simulink model "LinearRegressorIP"  (R2022b)
settings: Solver=VariableStepAuto  StartTime=0.0  StopTime=StopTime  RelTol=1e-3
values from neighbouring files (symbols this model uses):
  ADC_SampleTime = 1/ADC_Freq    (= 1e-06)    [LR_Init.m]
  Harmonics_Power = 1/2    (= 0.5)    [LR_Init.m]
  Noise_SampleTime = ADC_SampleTime    (= 1e-06)    [LR_Init.m]
  Noise_Source = 4    [LR_Init.m]
  Signal_Amp = 35    [LR_Init.m]
  Signal_Freq = 333    [LR_Init.m]
  Signal_Phase = pi/2    (= 1.57079632679)    [LR_Init.m]
  Spike_Level_min = 10    [LR_Init.m]
libraries: simulink x2
settings Model: Creator=Admin  LastModifiedBy=Admin

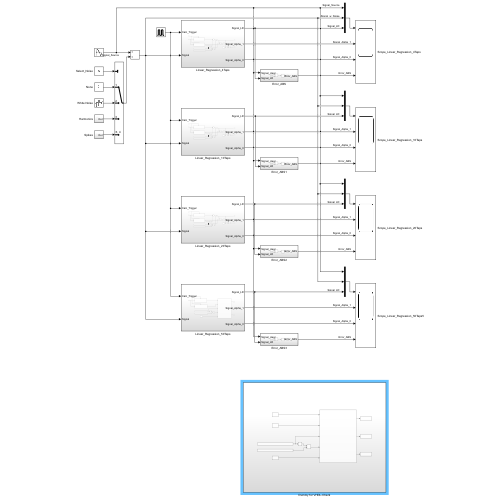
[thumbnail: Simulink's stored preview of the top-level diagram]
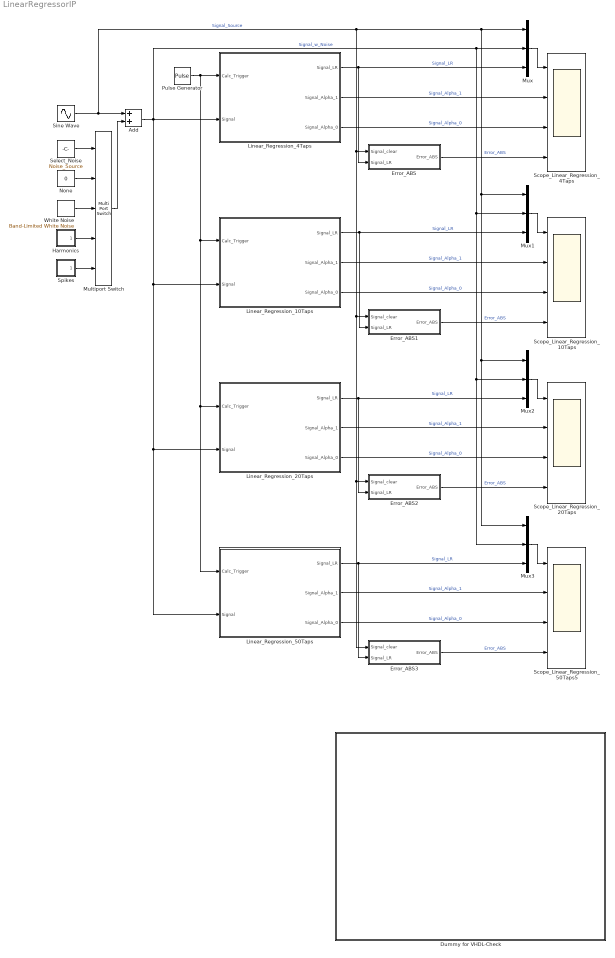
== system LinearRegressorIP ==
  Add : Sum
  Dummy for VHDL-Check : Subsystem
  Error_ABS : Subsystem
  Error_ABS1 : Subsystem
  Error_ABS2 : Subsystem
  Error_ABS3 : Subsystem
  Harmonics : Subsystem
  Linear_Regression_10Taps : Subsystem
  Linear_Regression_20Taps : Subsystem
  Linear_Regression_4Taps : Subsystem
  Linear_Regression_50Taps : Subsystem
  Multiport Switch : MultiPortSwitch  Inputs=4  SaturateOnIntegerOverflow=off  InputSameDT=off
  Mux{,1..3} (4 alike) : Mux  Inputs=3
  None : Constant  Value=0
  Pulse Generator : DiscretePulseGenerator  PulseType=Time based  Period=ADC_SampleTime  PulseWidth=50
  Scope_Linear_Regression_10Taps : Scope  NumInputPorts=4
  Scope_Linear_Regression_20Taps : Scope  NumInputPorts=4
  Scope_Linear_Regression_4Taps : Scope  NumInputPorts=4
  Scope_Linear_Regression_50Taps5 : Scope  NumInputPorts=4
  Select_Noise : Constant  Value=Noise_Source
  Sine Wave : Sin  Amplitude=Signal_Amp  Frequency=Signal_Freq*2*pi  Phase=Signal_Phase  SampleTime=0
  Spikes : Subsystem
  White Noise : simulink/Sources/Band-Limited White Noise  Cov=Noise_Power  Ts=Noise_SampleTime  seed=Noise_Seed
  wires:
  Pulse Generator/1 -> Linear_Regression_4Taps/1(Calc_Trigger), Linear_Regression_20Taps/1(Calc_Trigger), Linear_Regression_50Taps/1(Calc_Trigger), Linear_Regression_10Taps/1(Calc_Trigger)
  Sine Wave/1 -> Mux/1, Mux2/1, Mux3/1, Mux1/1, Error_ABS1/1(Signal_clear), Error_ABS3/1(Signal_clear), Error_ABS2/1(Signal_clear), Error_ABS/1(Signal_clear), Add/1  "Signal_Source"
  Multiport Switch/1 -> Add/2
  Add/1 -> Linear_Regression_4Taps/2(Signal), Linear_Regression_50Taps/2(Signal), Linear_Regression_20Taps/2(Signal), Linear_Regression_10Taps/2(Signal), Mux3/2, Mux2/2, Mux1/2, Mux/2  "Signal_w_Noise"
  Linear_Regression_4Taps/1(Signal_LR) -> Error_ABS/2(Signal_LR), Mux/3  "Signal_LR"
  Mux/1 -> Scope_Linear_Regression_4Taps/1
  Linear_Regression_4Taps/2(Signal_Alpha_1) -> Scope_Linear_Regression_4Taps/2  "Signal_Alpha_1"
  Linear_Regression_4Taps/3(Signal_Alpha_0) -> Scope_Linear_Regression_4Taps/3  "Signal_Alpha_0"
  Linear_Regression_10Taps/3(Signal_Alpha_0) -> Scope_Linear_Regression_10Taps/3  "Signal_Alpha_0"
  Linear_Regression_10Taps/2(Signal_Alpha_1) -> Scope_Linear_Regression_10Taps/2  "Signal_Alpha_1"
  Mux1/1 -> Scope_Linear_Regression_10Taps/1
  Linear_Regression_10Taps/1(Signal_LR) -> Error_ABS1/2(Signal_LR), Mux1/3  "Signal_LR"
  Mux2/1 -> Scope_Linear_Regression_20Taps/1
  Linear_Regression_20Taps/3(Signal_Alpha_0) -> Scope_Linear_Regression_20Taps/3  "Signal_Alpha_0"
  Linear_Regression_20Taps/2(Signal_Alpha_1) -> Scope_Linear_Regression_20Taps/2  "Signal_Alpha_1"
  Linear_Regression_20Taps/1(Signal_LR) -> Error_ABS2/2(Signal_LR), Mux2/3  "Signal_LR"
  Linear_Regression_50Taps/2(Signal_Alpha_1) -> Scope_Linear_Regression_50Taps5/2  "Signal_Alpha_1"
  Linear_Regression_50Taps/1(Signal_LR) -> Error_ABS3/2(Signal_LR), Mux3/3  "Signal_LR"
  Mux3/1 -> Scope_Linear_Regression_50Taps5/1
  Linear_Regression_50Taps/3(Signal_Alpha_0) -> Scope_Linear_Regression_50Taps5/3  "Signal_Alpha_0"
  Error_ABS/1(Error_ABS) -> Scope_Linear_Regression_4Taps/4  "Error_ABS"
  Error_ABS1/1(Error_ABS) -> Scope_Linear_Regression_10Taps/4  "Error_ABS"
  Error_ABS2/1(Error_ABS) -> Scope_Linear_Regression_20Taps/4  "Error_ABS"
  Error_ABS3/1(Error_ABS) -> Scope_Linear_Regression_50Taps5/4  "Error_ABS"
  Select_Noise/1 -> Multiport Switch/1
  None/1 -> Multiport Switch/2
  White Noise/1 -> Multiport Switch/3
  Harmonics/1(Out) -> Multiport Switch/4
  Spikes/1(Out) -> Multiport Switch/5

== system LinearRegressorIP/Dummy for VHDL-Check ==
  Constant : Constant  Value=50
  Constant3 : Constant  Value=25.5
  Constant4 : Constant  Value=858.5
  Constant5 : Constant
  LR_Calcer : Subsystem
  Pulse Generator : DiscretePulseGenerator  PulseType=Time based  Period=ADC_SampleTime  PulseWidth=50
  Running_mean_Window_50_Signal : Subsystem
  Running_mean_Window_50_SignalTimesSample : Subsystem
  Scope : Scope
  Scope1 : Scope
  Scope2 : Scope  NumInputPorts=3
  Square : Math  Operator=square
  Subtract1 : Sum  Inputs=-+
  wires:
  Subtract1/1 -> LR_Calcer/4(FaktorCalcAlpha1)
  Constant/1 -> LR_Calcer/5(Tabs)
  Constant4/1 -> Subtract1/2
  Constant3/1 -> Square/1, LR_Calcer/3(samples_mean)
  Square/1 -> Subtract1/1
  LR_Calcer/3(Signal_LR) -> Scope2/3  "Signal_LR"
  Running_mean_Window_50_SignalTimesSample/1(Signal_Output_Mean) -> LR_Calcer/1(RMW_SignalTimesSample), Scope/1
  Running_mean_Window_50_Signal/1(Signal_Output_Mean) -> LR_Calcer/2(RMW_Signal), Scope1/1
  Pulse Generator/1 -> Running_mean_Window_50_Signal/Trigger, Running_mean_Window_50_SignalTimesSample/Trigger
  Constant5/1 -> Running_mean_Window_50_SignalTimesSample/1(Signal_Input), Running_mean_Window_50_Signal/1(Signal_Input)
  LR_Calcer/1(Alpha_1) -> Scope2/1  "Alpha_1"
  LR_Calcer/2(Alpha_0) -> Scope2/2  "Alpha_0"

== system LinearRegressorIP/Error_ABS ==
  Signal_clear : Inport
  Signal_LR : Inport  Port=2
  Abs : Abs  SaturateOnIntegerOverflow=off
  Subtract : Sum  Inputs=+-
  Error_ABS : Outport
  wires:
  Abs/1 -> Error_ABS/1
  Subtract/1 -> Abs/1
  Signal_clear/1 -> Subtract/1
  Signal_LR/1 -> Subtract/2

== system LinearRegressorIP/Error_ABS1 ==
  Signal_clear : Inport
  Signal_LR : Inport  Port=2
  Abs : Abs  SaturateOnIntegerOverflow=off
  Subtract : Sum  Inputs=+-
  Error_ABS : Outport
  wires:
  Signal_LR/1 -> Subtract/2
  Signal_clear/1 -> Subtract/1
  Subtract/1 -> Abs/1
  Abs/1 -> Error_ABS/1

== system LinearRegressorIP/Error_ABS2 ==
  Signal_clear : Inport
  Signal_LR : Inport  Port=2
  Abs : Abs  SaturateOnIntegerOverflow=off
  Subtract : Sum  Inputs=+-
  Error_ABS : Outport
  wires:
  Abs/1 -> Error_ABS/1
  Subtract/1 -> Abs/1
  Signal_clear/1 -> Subtract/1
  Signal_LR/1 -> Subtract/2

== system LinearRegressorIP/Error_ABS3 ==
  Signal_clear : Inport
  Signal_LR : Inport  Port=2
  Abs : Abs  SaturateOnIntegerOverflow=off
  Subtract : Sum  Inputs=+-
  Error_ABS : Outport
  wires:
  Signal_LR/1 -> Subtract/2
  Signal_clear/1 -> Subtract/1
  Subtract/1 -> Abs/1
  Abs/1 -> Error_ABS/1

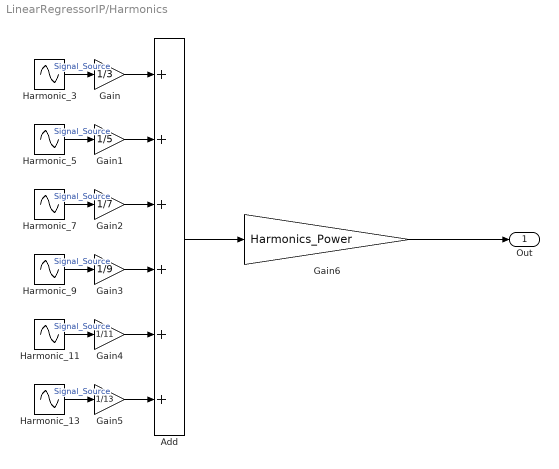
== system LinearRegressorIP/Harmonics ==
  Add : Sum  Inputs=++++++
  Gain : Gain  Gain=1/3
  Gain1 : Gain  Gain=1/5
  Gain2 : Gain  Gain=1/7
  Gain3 : Gain  Gain=1/9
  Gain4 : Gain  Gain=1/11
  Gain5 : Gain  Gain=1/13
  Gain6 : Gain  Gain=Harmonics_Power
  Harmonic_11 : Sin  Amplitude=Signal_Amp  Frequency=Signal_Freq*2*pi*11  Phase=Signal_Phase  SampleTime=0
  Harmonic_13 : Sin  Amplitude=Signal_Amp  Frequency=Signal_Freq*2*pi*13  Phase=Signal_Phase  SampleTime=0
  Harmonic_3 : Sin  Amplitude=Signal_Amp  Frequency=Signal_Freq*2*pi*3  Phase=Signal_Phase  SampleTime=0
  Harmonic_5 : Sin  Amplitude=Signal_Amp  Frequency=Signal_Freq*2*pi*5  Phase=Signal_Phase  SampleTime=0
  Harmonic_7 : Sin  Amplitude=Signal_Amp  Frequency=Signal_Freq*2*pi*7  Phase=Signal_Phase  SampleTime=0
  Harmonic_9 : Sin  Amplitude=Signal_Amp  Frequency=Signal_Freq*2*pi*9  Phase=Signal_Phase  SampleTime=0
  Out : Outport
  wires:
  Gain/1 -> Add/1
  Add/1 -> Gain6/1
  Gain6/1 -> Out/1
  Harmonic_5/1 -> Gain1/1  "Signal_Source"
  Harmonic_7/1 -> Gain2/1  "Signal_Source"
  Harmonic_9/1 -> Gain3/1  "Signal_Source"
  Harmonic_11/1 -> Gain4/1  "Signal_Source"
  Harmonic_13/1 -> Gain5/1  "Signal_Source"
  Gain5/1 -> Add/6
  Gain4/1 -> Add/5
  Gain3/1 -> Add/4
  Gain2/1 -> Add/3
  Gain1/1 -> Add/2
  Harmonic_3/1 -> Gain/1  "Signal_Source"

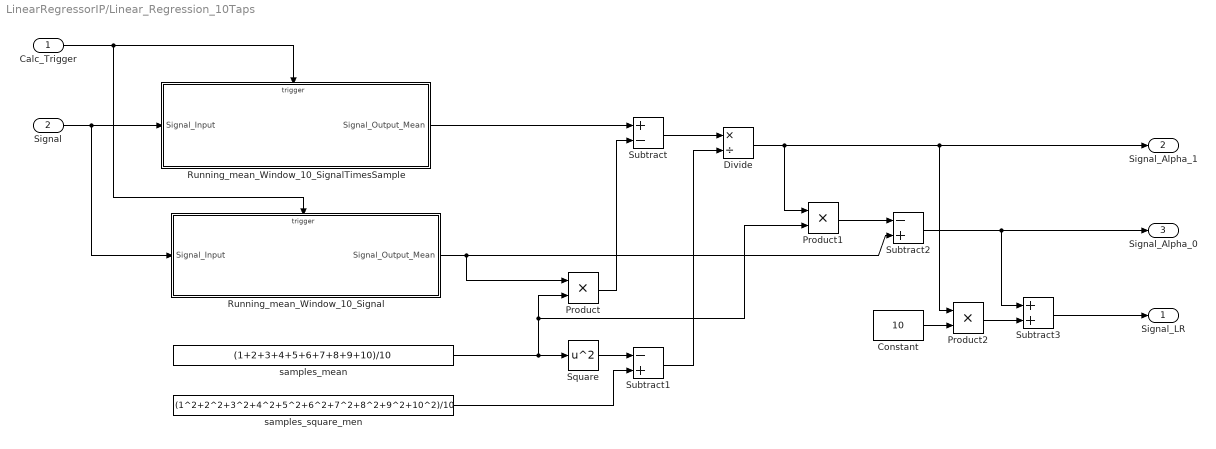
== system LinearRegressorIP/Linear_Regression_10Taps ==
  Calc_Trigger : Inport
  Signal : Inport  Port=2
  Constant : Constant  Value=10
  Divide : Product  Inputs=*/
  Product : Product
  Product1 : Product
  Product2 : Product
  Running_mean_Window_10_Signal : Subsystem
  Running_mean_Window_10_SignalTimesSample : Subsystem
  Square : Math  Operator=square
  Subtract : Sum  Inputs=+-
  Subtract1 : Sum  Inputs=-+
  Subtract2 : Sum  Inputs=-+
  Subtract3 : Sum
  samples_mean : Constant  Value=(1+2+3+4+5+6+7+8+9+10)/10
  samples_square_men : Constant  Value=(1^2+2^2+3^2+4^2+5^2+6^2+7^2+8^2+9^2+10^2)/10
  Signal_LR : Outport
  Signal_Alpha_1 : Outport  Port=2
  Signal_Alpha_0 : Outport  Port=3
  wires:
  samples_mean/1 -> Product1/2, Product/2, Square/1
  Subtract/1 -> Divide/1
  Square/1 -> Subtract1/1
  Divide/1 -> Signal_Alpha_1/1, Product2/1, Product1/1
  Product2/1 -> Subtract3/2
  Constant/1 -> Product2/2
  Subtract1/1 -> Divide/2
  Signal/1 -> Running_mean_Window_10_SignalTimesSample/1(Signal_Input), Running_mean_Window_10_Signal/1(Signal_Input)
  samples_square_men/1 -> Subtract1/2
  Calc_Trigger/1 -> Running_mean_Window_10_SignalTimesSample/Trigger, Running_mean_Window_10_Signal/Trigger
  Running_mean_Window_10_Signal/1(Signal_Output_Mean) -> Subtract2/2, Product/1
  Subtract2/1 -> Signal_Alpha_0/1, Subtract3/1
  Product1/1 -> Subtract2/1
  Subtract3/1 -> Signal_LR/1
  Product/1 -> Subtract/2
  Running_mean_Window_10_SignalTimesSample/1(Signal_Output_Mean) -> Subtract/1

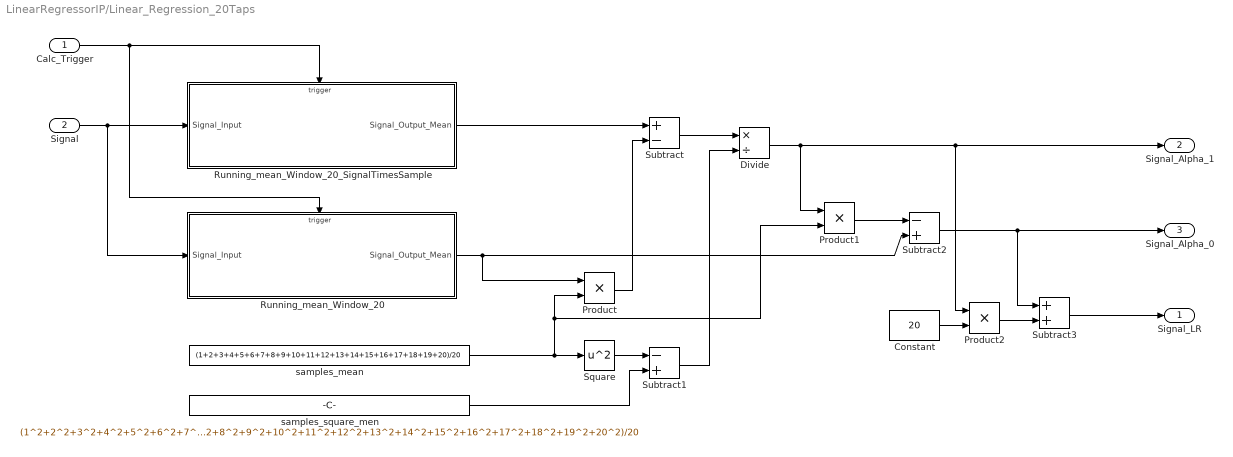
== system LinearRegressorIP/Linear_Regression_20Taps ==
  Calc_Trigger : Inport
  Signal : Inport  Port=2
  Constant : Constant  Value=20
  Divide : Product  Inputs=*/
  Product : Product
  Product1 : Product
  Product2 : Product
  Running_mean_Window_20 : Subsystem
  Running_mean_Window_20_SignalTimesSample : Subsystem
  Square : Math  Operator=square
  Subtract : Sum  Inputs=+-
  Subtract1 : Sum  Inputs=-+
  Subtract2 : Sum  Inputs=-+
  Subtract3 : Sum
  samples_mean : Constant  Value=(1+2+3+4+5+6+7+8+9+10+11+12+13+14+15+16+17+18+19+20)/20
  samples_square_men : Constant  Value=(1^2+2^2+3^2+4^2+5^2+6^2+7^2+8^2+9^2+10^2+11^2+12^2+13^2+14^2+15^2+16^2+17^2+18^2+19^2+20^2)/20
  Signal_LR : Outport
  Signal_Alpha_1 : Outport  Port=2
  Signal_Alpha_0 : Outport  Port=3
  wires:
  Running_mean_Window_20_SignalTimesSample/1(Signal_Output_Mean) -> Subtract/1
  Product/1 -> Subtract/2
  Subtract3/1 -> Signal_LR/1
  Product1/1 -> Subtract2/1
  Subtract2/1 -> Subtract3/1, Signal_Alpha_0/1
  Running_mean_Window_20/1(Signal_Output_Mean) -> Product/1, Subtract2/2
  Calc_Trigger/1 -> Running_mean_Window_20/Trigger, Running_mean_Window_20_SignalTimesSample/Trigger
  samples_square_men/1 -> Subtract1/2
  Signal/1 -> Running_mean_Window_20/1(Signal_Input), Running_mean_Window_20_SignalTimesSample/1(Signal_Input)
  Subtract1/1 -> Divide/2
  Constant/1 -> Product2/2
  Product2/1 -> Subtract3/2
  Divide/1 -> Product1/1, Product2/1, Signal_Alpha_1/1
  Square/1 -> Subtract1/1
  Subtract/1 -> Divide/1
  samples_mean/1 -> Square/1, Product/2, Product1/2

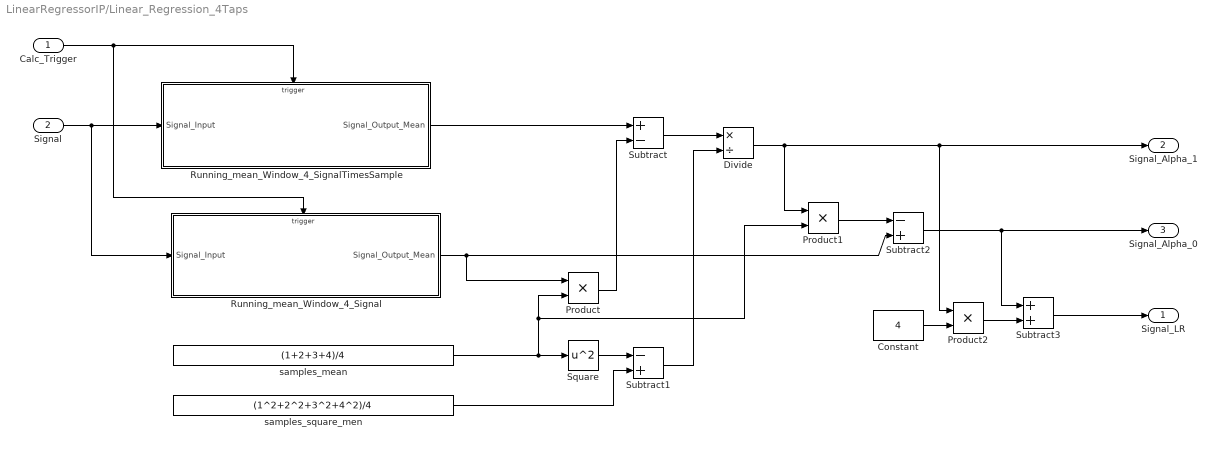
== system LinearRegressorIP/Linear_Regression_4Taps ==
  Calc_Trigger : Inport
  Signal : Inport  Port=2
  Constant : Constant  Value=4
  Divide : Product  Inputs=*/
  Product : Product
  Product1 : Product
  Product2 : Product
  Running_mean_Window_4_Signal : Subsystem
  Running_mean_Window_4_SignalTimesSample : Subsystem
  Square : Math  Operator=square
  Subtract : Sum  Inputs=+-
  Subtract1 : Sum  Inputs=-+
  Subtract2 : Sum  Inputs=-+
  Subtract3 : Sum
  samples_mean : Constant  Value=(1+2+3+4)/4
  samples_square_men : Constant  Value=(1^2+2^2+3^2+4^2)/4
  Signal_LR : Outport
  Signal_Alpha_1 : Outport  Port=2
  Signal_Alpha_0 : Outport  Port=3
  wires:
  Running_mean_Window_4_SignalTimesSample/1(Signal_Output_Mean) -> Subtract/1
  Product/1 -> Subtract/2
  Subtract3/1 -> Signal_LR/1
  Product1/1 -> Subtract2/1
  Subtract2/1 -> Subtract3/1, Signal_Alpha_0/1
  Running_mean_Window_4_Signal/1(Signal_Output_Mean) -> Product/1, Subtract2/2
  Calc_Trigger/1 -> Running_mean_Window_4_Signal/Trigger, Running_mean_Window_4_SignalTimesSample/Trigger
  samples_square_men/1 -> Subtract1/2
  Signal/1 -> Running_mean_Window_4_Signal/1(Signal_Input), Running_mean_Window_4_SignalTimesSample/1(Signal_Input)
  Subtract1/1 -> Divide/2
  Constant/1 -> Product2/2
  Product2/1 -> Subtract3/2
  Divide/1 -> Product1/1, Product2/1, Signal_Alpha_1/1
  Square/1 -> Subtract1/1
  Subtract/1 -> Divide/1
  samples_mean/1 -> Square/1, Product/2, Product1/2

== system LinearRegressorIP/Linear_Regression_50Taps ==
  Calc_Trigger : Inport
  Signal : Inport  Port=2
  Constant : Constant  Value=50
  LR_Calcer : Subsystem
  Running_mean_Window_50_Signal : Subsystem
  Running_mean_Window_50_SignalTimesSample : Subsystem
  Square : Math  Operator=square
  Subtract1 : Sum  Inputs=-+
  samples_mean : Constant  Value=25.5
  samples_square_men : Constant  Value=858.5
  Signal_LR : Outport
  Signal_Alpha_1 : Outport  Port=2
  Signal_Alpha_0 : Outport  Port=3
  wires:
  samples_mean/1 -> LR_Calcer/3(samples_mean), Square/1
  Square/1 -> Subtract1/1
  Signal/1 -> Running_mean_Window_50_Signal/1(Signal_Input), Running_mean_Window_50_SignalTimesSample/1(Signal_Input)
  samples_square_men/1 -> Subtract1/2
  Calc_Trigger/1 -> Running_mean_Window_50_Signal/Trigger, Running_mean_Window_50_SignalTimesSample/Trigger
  Running_mean_Window_50_SignalTimesSample/1(Signal_Output_Mean) -> LR_Calcer/1(RMW_SignalTimesSample)
  Running_mean_Window_50_Signal/1(Signal_Output_Mean) -> LR_Calcer/2(RMW_SignalT)
  Subtract1/1 -> LR_Calcer/4(FaktorCalcAlpha1)
  LR_Calcer/1(Alpha_1) -> Signal_Alpha_1/1
  LR_Calcer/2(Alpha_0) -> Signal_Alpha_0/1
  LR_Calcer/3(Signal_LR) -> Signal_LR/1
  Constant/1 -> LR_Calcer/5(Tabs)

== system LinearRegressorIP/Spikes ==
  Abs : Abs  SaturateOnIntegerOverflow=off
  Constant : Constant  Value=Spike_Level_min
  Constant1 : Constant  Value=0
  GreaterThan : RelationalOperator  Operator=>  OutDataTypeStr=boolean  RndMeth=Simplest  InputSameDT=off
  Switch : Switch  Criteria=u2 > Threshold  SaturateOnIntegerOverflow=off  InputSameDT=off
  White Noise : simulink/Sources/Band-Limited White Noise  Cov=Noise_Power  Ts=Noise_SampleTime  seed=Noise_Seed
  Out : Outport
  wires:
  Constant/1 -> GreaterThan/2
  White Noise/1 -> Abs/1, Switch/1
  GreaterThan/1 -> Switch/2
  Constant1/1 -> Switch/3
  Switch/1 -> Out/1
  Abs/1 -> GreaterThan/1

== system LinearRegressorIP/Dummy for VHDL-Check/LR_Calcer ==
  RMW_SignalTimesSample : Inport
  RMW_Signal : Inport  Port=2
  samples_mean : Inport  Port=3
  FaktorCalcAlpha1 : Inport  Port=4
  Tabs : Inport  Port=5
  Divide : Product  Inputs=*/
  Product : Product
  Product1 : Product
  Product2 : Product
  Subtract : Sum  Inputs=+-
  Subtract2 : Sum  Inputs=-+
  Subtract3 : Sum
  Alpha_1 : Outport
  Alpha_0 : Outport  Port=2
  Signal_LR : Outport  Port=3
  wires:
  samples_mean/1 -> Product1/2, Product/2
  RMW_Signal/1 -> Subtract2/2, Product/1
  Tabs/1 -> Product2/2
  Divide/1 -> Alpha_1/1, Product2/1, Product1/1
  Product1/1 -> Subtract2/1
  Subtract/1 -> Divide/1
  Subtract2/1 -> Alpha_0/1, Subtract3/1
  Product/1 -> Subtract/2
  RMW_SignalTimesSample/1 -> Subtract/1
  Product2/1 -> Subtract3/2
  FaktorCalcAlpha1/1 -> Divide/2
  Subtract3/1 -> Signal_LR/1

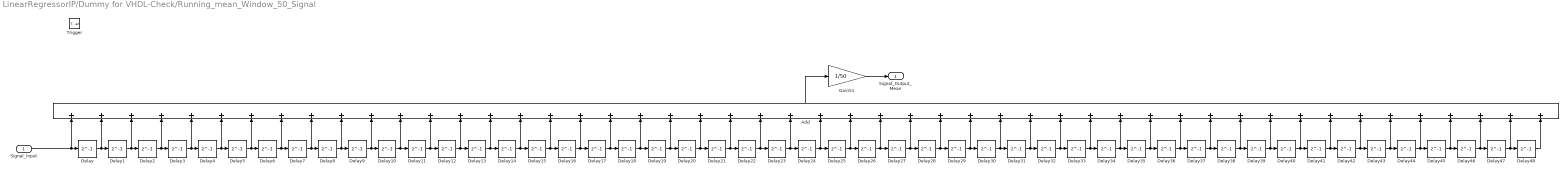
== system LinearRegressorIP/Dummy for VHDL-Check/Running_mean_Window_50_Signal ==
  Signal_Input : Inport
  Trigger : TriggerPort  VariantControl=(inherit)  PortDimensions=1
  Add : Sum  Inputs=++++++++++++++++++++++++++++++++++++++++++++++++++
  Delay{,1..48} (49 alike) : Delay  DelayLength=1
  Gain51 : Gain  Gain=1/50
  Signal_Output_Mean : Outport
  wires:
  Gain51/1 -> Signal_Output_Mean/1
  Delay30/1 -> Add/32, Delay31/1
  Delay28/1 -> Add/30, Delay29/1
  Delay27/1 -> Add/29, Delay28/1
  Delay48/1 -> Add/50
  Delay26/1 -> Add/28, Delay27/1
  Delay7/1 -> Add/9, Delay8/1
  Delay29/1 -> Add/31, Delay30/1
  Delay33/1 -> Add/35, Delay34/1
  Delay24/1 -> Add/26, Delay25/1
  Signal_Input/1 -> Add/1, Delay/1
  Delay23/1 -> Add/25, Delay24/1
  Delay22/1 -> Add/24, Delay23/1
  Delay18/1 -> Add/20, Delay19/1
  Delay21/1 -> Add/23, Delay22/1
  Delay19/1 -> Add/21, Delay20/1
  Delay17/1 -> Add/19, Delay18/1
  Delay/1 -> Add/2, Delay1/1
  Delay9/1 -> Add/11, Delay10/1
  Delay16/1 -> Add/18, Delay17/1
  Delay11/1 -> Add/13, Delay12/1
  Delay12/1 -> Add/14, Delay13/1
  Delay41/1 -> Add/43, Delay42/1
  Delay38/1 -> Add/40, Delay39/1
  Delay40/1 -> Add/42, Delay41/1
  Delay34/1 -> Add/36, Delay35/1
  Delay36/1 -> Add/38, Delay37/1
  Delay35/1 -> Add/37, Delay36/1
  Delay43/1 -> Add/45, Delay44/1
  Delay39/1 -> Add/41, Delay40/1
  Delay32/1 -> Add/34, Delay33/1
  Delay2/1 -> Add/4, Delay3/1
  Delay37/1 -> Add/39, Delay38/1
  Delay20/1 -> Add/22, Delay21/1
  Delay13/1 -> Add/15, Delay14/1
  Add/1 -> Gain51/1
  Delay8/1 -> Add/10, Delay9/1
  Delay6/1 -> Add/8, Delay7/1
  Delay4/1 -> Add/6, Delay5/1
  Delay5/1 -> Add/7, Delay6/1
  Delay3/1 -> Add/5, Delay4/1
  Delay1/1 -> Add/3, Delay2/1
  Delay42/1 -> Add/44, Delay43/1
  Delay25/1 -> Add/27, Delay26/1
  Delay44/1 -> Add/46, Delay45/1
  Delay31/1 -> Add/33, Delay32/1
  Delay14/1 -> Add/16, Delay15/1
  Delay46/1 -> Add/48, Delay47/1
  Delay10/1 -> Add/12, Delay11/1
  Delay45/1 -> Add/47, Delay46/1
  Delay47/1 -> Add/49, Delay48/1
  Delay15/1 -> Add/17, Delay16/1

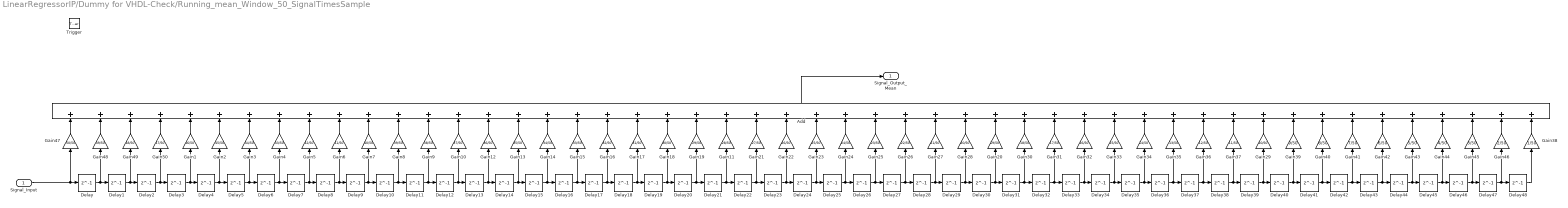
== system LinearRegressorIP/Dummy for VHDL-Check/Running_mean_Window_50_SignalTimesSample ==
  Signal_Input : Inport
  Trigger : TriggerPort  VariantControl=(inherit)  PortDimensions=1
  Add : Sum  Inputs=++++++++++++++++++++++++++++++++++++++++++++++++++
  Delay{,1..48} (49 alike) : Delay  DelayLength=1
  Gain1 : Gain  Gain=46/50
  Gain10 : Gain  Gain=37/50
  Gain11 : Gain  Gain=28/50
  Gain12 : Gain  Gain=36/50
  Gain13 : Gain  Gain=35/50
  Gain14 : Gain  Gain=34/50
  Gain15 : Gain  Gain=33/50
  Gain16 : Gain  Gain=32/50
  Gain17 : Gain  Gain=31/50
  Gain18 : Gain  Gain=30/50
  Gain19 : Gain  Gain=29/50
  Gain2 : Gain  Gain=45/50
  Gain20 : Gain  Gain=19/50
  Gain21 : Gain  Gain=27/50
  Gain22 : Gain  Gain=26/50
  Gain23 : Gain  Gain=25/50
  Gain24 : Gain  Gain=24/50
  Gain25 : Gain  Gain=23/50
  Gain26 : Gain  Gain=22/50
  Gain27 : Gain  Gain=21/50
  Gain28 : Gain  Gain=20/50
  Gain29 : Gain  Gain=10/50
  Gain3 : Gain  Gain=44/50
  Gain30 : Gain  Gain=18/50
  Gain31 : Gain  Gain=17/50
  Gain32 : Gain  Gain=16/50
  Gain33 : Gain  Gain=15/50
  Gain34 : Gain  Gain=14/50
  Gain35 : Gain  Gain=13/50
  Gain36 : Gain  Gain=12/50
  Gain37 : Gain  Gain=11/50
  Gain38 : Gain  Gain=1/50
  Gain39 : Gain  Gain=9/50
  Gain4 : Gain  Gain=43/50
  Gain40 : Gain  Gain=8/50
  Gain41 : Gain  Gain=7/50
  Gain42 : Gain  Gain=6/50
  Gain43 : Gain  Gain=5/50
  Gain44 : Gain  Gain=4/50
  Gain45 : Gain  Gain=3/50
  Gain46 : Gain  Gain=2/50
  Gain47 : Gain  Gain=50/50
  Gain48 : Gain  Gain=49/50
  Gain49 : Gain  Gain=48/50
  Gain5 : Gain  Gain=42/50
  Gain50 : Gain  Gain=47/50
  Gain6 : Gain  Gain=41/50
  Gain7 : Gain  Gain=40/50
  Gain8 : Gain  Gain=39/50
  Gain9 : Gain  Gain=38/50
  Signal_Output_Mean : Outport
  wires:
  Signal_Input/1 -> Gain47/1, Delay/1
  Delay8/1 -> Gain6/1, Delay9/1
  Delay5/1 -> Gain3/1, Delay6/1
  Delay4/1 -> Gain2/1, Delay5/1
  Delay/1 -> Gain48/1, Delay1/1
  Delay3/1 -> Gain1/1, Delay4/1
  Delay6/1 -> Gain4/1, Delay7/1
  Delay1/1 -> Gain49/1, Delay2/1
  Delay2/1 -> Gain50/1, Delay3/1
  Delay7/1 -> Gain5/1, Delay8/1
  Gain1/1 -> Add/5
  Gain2/1 -> Add/6
  Gain3/1 -> Add/7
  Gain4/1 -> Add/8
  Gain5/1 -> Add/9
  Gain6/1 -> Add/10
  Gain7/1 -> Add/11
  Gain8/1 -> Add/12
  Gain9/1 -> Add/13
  Gain10/1 -> Add/14
  Gain11/1 -> Add/23
  Gain13/1 -> Add/16
  Gain19/1 -> Add/22
  Delay16/1 -> Gain15/1, Delay17/1
  Gain18/1 -> Add/21
  Gain14/1 -> Add/17
  Delay12/1 -> Gain10/1, Delay13/1
  Gain16/1 -> Add/19
  Gain15/1 -> Add/18
  Gain17/1 -> Add/20
  Delay11/1 -> Gain9/1, Delay12/1
  Delay10/1 -> Gain8/1, Delay11/1
  Delay15/1 -> Gain14/1, Delay16/1
  Delay9/1 -> Gain7/1, Delay10/1
  Delay14/1 -> Gain13/1, Delay15/1
  Gain12/1 -> Add/15
  Delay13/1 -> Gain12/1, Delay14/1
  Delay17/1 -> Gain16/1, Delay18/1
  Gain20/1 -> Add/32
  Gain22/1 -> Add/25
  Gain28/1 -> Add/31
  Delay25/1 -> Gain24/1, Delay26/1
  Gain27/1 -> Add/30
  Gain23/1 -> Add/26
  Delay21/1 -> Gain11/1, Delay22/1
  Gain25/1 -> Add/28
  Gain24/1 -> Add/27
  Gain26/1 -> Add/29
  Delay20/1 -> Gain19/1, Delay21/1
  Delay19/1 -> Gain18/1, Delay20/1
  Delay24/1 -> Gain23/1, Delay25/1
  Delay18/1 -> Gain17/1, Delay19/1
  Delay23/1 -> Gain22/1, Delay24/1
  Gain21/1 -> Add/24
  Delay22/1 -> Gain21/1, Delay23/1
  Delay26/1 -> Gain25/1, Delay27/1
  Gain29/1 -> Add/41
  Gain31/1 -> Add/34
  Gain37/1 -> Add/40
  Delay34/1 -> Gain33/1, Delay35/1
  Gain36/1 -> Add/39
  Gain32/1 -> Add/35
  Delay30/1 -> Gain20/1, Delay31/1
  Gain34/1 -> Add/37
  Gain33/1 -> Add/36
  Gain35/1 -> Add/38
  Delay29/1 -> Gain28/1, Delay30/1
  Delay28/1 -> Gain27/1, Delay29/1
  Delay33/1 -> Gain32/1, Delay34/1
  Delay27/1 -> Gain26/1, Delay28/1
  Delay32/1 -> Gain31/1, Delay33/1
  Gain30/1 -> Add/33
  Delay31/1 -> Gain30/1, Delay32/1
  Delay35/1 -> Gain34/1, Delay36/1
  Gain38/1 -> Add/50
  Gain40/1 -> Add/43
  Gain46/1 -> Add/49
  Delay43/1 -> Gain42/1, Delay44/1
  Gain45/1 -> Add/48
  Gain41/1 -> Add/44
  Delay39/1 -> Gain29/1, Delay40/1
  Gain43/1 -> Add/46
  Gain42/1 -> Add/45
  Gain44/1 -> Add/47
  Delay38/1 -> Gain37/1, Delay39/1
  Delay37/1 -> Gain36/1, Delay38/1
  Delay42/1 -> Gain41/1, Delay43/1
  Delay36/1 -> Gain35/1, Delay37/1
  Delay41/1 -> Gain40/1, Delay42/1
  Gain39/1 -> Add/42
  Delay40/1 -> Gain39/1, Delay41/1
  Delay44/1 -> Gain43/1, Delay45/1
  Delay48/1 -> Gain38/1
  Delay45/1 -> Gain44/1, Delay46/1
  Delay46/1 -> Gain45/1, Delay47/1
  Delay47/1 -> Gain46/1, Delay48/1
  Gain50/1 -> Add/4
  Gain49/1 -> Add/3
  Gain48/1 -> Add/2
  Gain47/1 -> Add/1
  Add/1 -> Signal_Output_Mean/1

== system LinearRegressorIP/Linear_Regression_10Taps/Running_mean_Window_10_Signal ==
  Signal_Input : Inport
  Trigger : TriggerPort  VariantControl=(inherit)  PortDimensions=1
  Add : Sum  Inputs=++++++++++
  Delay{,1..8} (9 alike) : Delay  DelayLength=1
  Gain : Gain  Gain=1/10
  Signal_Output_Mean : Outport
  wires:
  Delay7/1 -> Add/9, Delay8/1
  Delay2/1 -> Add/4, Delay3/1
  Delay1/1 -> Add/3, Delay2/1
  Delay6/1 -> Add/8, Delay7/1
  Delay3/1 -> Add/5, Delay4/1
  Add/1 -> Gain/1
  Delay/1 -> Add/2, Delay1/1
  Delay4/1 -> Add/6, Delay5/1
  Delay5/1 -> Add/7, Delay6/1
  Delay8/1 -> Add/10
  Signal_Input/1 -> Add/1, Delay/1
  Gain/1 -> Signal_Output_Mean/1

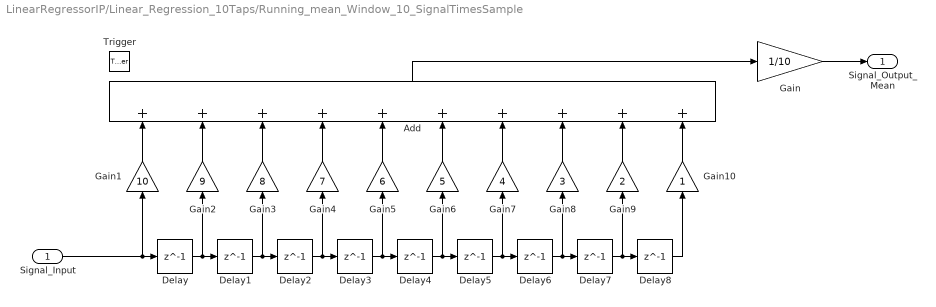
== system LinearRegressorIP/Linear_Regression_10Taps/Running_mean_Window_10_SignalTimesSample ==
  Signal_Input : Inport
  Trigger : TriggerPort  VariantControl=(inherit)  PortDimensions=1
  Add : Sum  Inputs=++++++++++
  Delay{,1..8} (9 alike) : Delay  DelayLength=1
  Gain : Gain  Gain=1/10
  Gain1 : Gain  Gain=10
  Gain10 : Gain
  Gain2 : Gain  Gain=9
  Gain3 : Gain  Gain=8
  Gain4 : Gain  Gain=7
  Gain5 : Gain  Gain=6
  Gain6 : Gain  Gain=5
  Gain7 : Gain  Gain=4
  Gain8 : Gain  Gain=3
  Gain9 : Gain  Gain=2
  Signal_Output_Mean : Outport
  wires:
  Gain/1 -> Signal_Output_Mean/1
  Signal_Input/1 -> Delay/1, Gain1/1
  Delay8/1 -> Gain10/1
  Delay5/1 -> Delay6/1, Gain7/1
  Delay4/1 -> Delay5/1, Gain6/1
  Delay/1 -> Delay1/1, Gain2/1
  Delay3/1 -> Delay4/1, Gain5/1
  Delay6/1 -> Delay7/1, Gain8/1
  Delay1/1 -> Delay2/1, Gain3/1
  Delay2/1 -> Delay3/1, Gain4/1
  Delay7/1 -> Delay8/1, Gain9/1
  Gain1/1 -> Add/1
  Gain2/1 -> Add/2
  Gain3/1 -> Add/3
  Gain4/1 -> Add/4
  Gain5/1 -> Add/5
  Gain6/1 -> Add/6
  Gain7/1 -> Add/7
  Gain8/1 -> Add/8
  Gain9/1 -> Add/9
  Gain10/1 -> Add/10
  Add/1 -> Gain/1

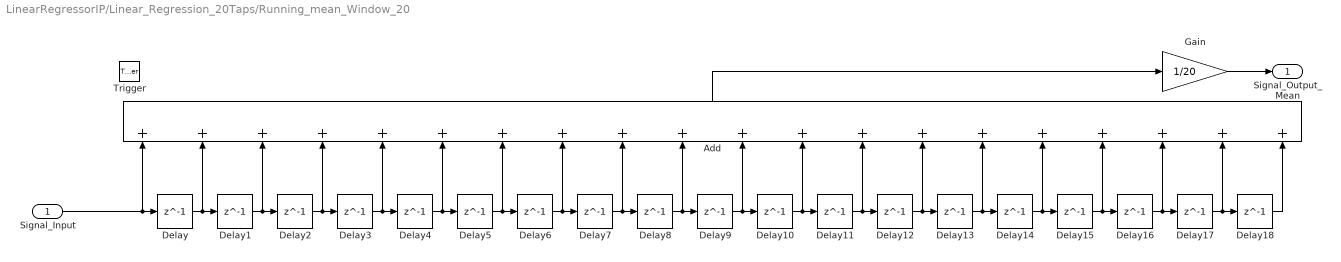
== system LinearRegressorIP/Linear_Regression_20Taps/Running_mean_Window_20 ==
  Signal_Input : Inport
  Trigger : TriggerPort  VariantControl=(inherit)  PortDimensions=1
  Add : Sum  Inputs=++++++++++++++++++++
  Delay{,1..18} (19 alike) : Delay  DelayLength=1
  Gain : Gain  Gain=1/20
  Signal_Output_Mean : Outport
  wires:
  Add/1 -> Gain/1
  Delay18/1 -> Add/20
  Delay13/1 -> Add/15, Delay14/1
  Delay16/1 -> Add/18, Delay17/1
  Delay14/1 -> Add/16, Delay15/1
  Delay15/1 -> Add/17, Delay16/1
  Delay17/1 -> Add/19, Delay18/1
  Delay11/1 -> Add/13, Delay12/1
  Delay9/1 -> Add/11, Delay10/1
  Delay10/1 -> Add/12, Delay11/1
  Delay12/1 -> Add/14, Delay13/1
  Gain/1 -> Signal_Output_Mean/1
  Signal_Input/1 -> Add/1, Delay/1
  Delay/1 -> Add/2, Delay1/1
  Delay1/1 -> Add/3, Delay2/1
  Delay2/1 -> Add/4, Delay3/1
  Delay3/1 -> Add/5, Delay4/1
  Delay4/1 -> Add/6, Delay5/1
  Delay5/1 -> Add/7, Delay6/1
  Delay6/1 -> Add/8, Delay7/1
  Delay7/1 -> Add/9, Delay8/1
  Delay8/1 -> Add/10, Delay9/1

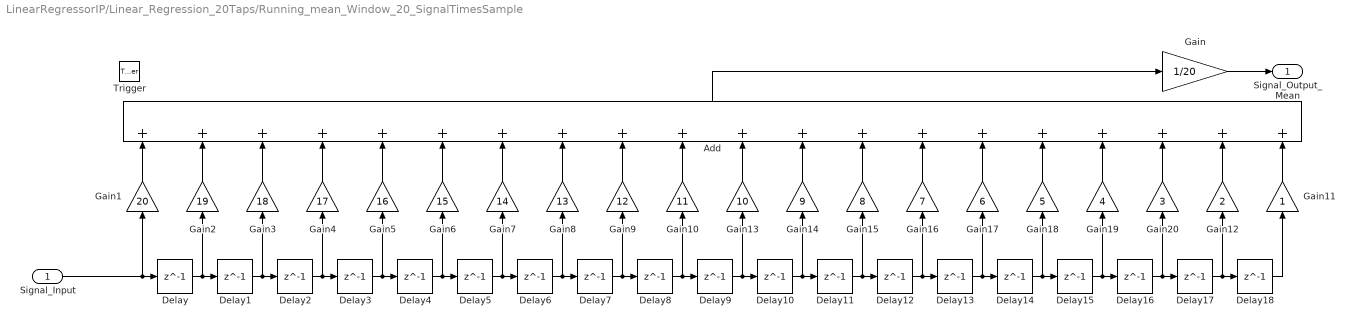
== system LinearRegressorIP/Linear_Regression_20Taps/Running_mean_Window_20_SignalTimesSample ==
  Signal_Input : Inport
  Trigger : TriggerPort  VariantControl=(inherit)  PortDimensions=1
  Add : Sum  Inputs=++++++++++++++++++++
  Delay{,1..18} (19 alike) : Delay  DelayLength=1
  Gain : Gain  Gain=1/20
  Gain1 : Gain  Gain=20
  Gain10 : Gain  Gain=11
  Gain11 : Gain
  Gain12 : Gain  Gain=2
  Gain13 : Gain  Gain=10
  Gain14 : Gain  Gain=9
  Gain15 : Gain  Gain=8
  Gain16 : Gain  Gain=7
  Gain17 : Gain  Gain=6
  Gain18 : Gain  Gain=5
  Gain19 : Gain  Gain=4
  Gain2 : Gain  Gain=19
  Gain20 : Gain  Gain=3
  Gain3 : Gain  Gain=18
  Gain4 : Gain  Gain=17
  Gain5 : Gain  Gain=16
  Gain6 : Gain  Gain=15
  Gain7 : Gain  Gain=14
  Gain8 : Gain  Gain=13
  Gain9 : Gain  Gain=12
  Signal_Output_Mean : Outport
  wires:
  Gain10/1 -> Add/10
  Gain9/1 -> Add/9
  Gain8/1 -> Add/8
  Gain7/1 -> Add/7
  Gain6/1 -> Add/6
  Gain5/1 -> Add/5
  Gain4/1 -> Add/4
  Gain3/1 -> Add/3
  Gain2/1 -> Add/2
  Gain1/1 -> Add/1
  Delay7/1 -> Gain9/1, Delay8/1
  Delay2/1 -> Gain4/1, Delay3/1
  Delay1/1 -> Gain3/1, Delay2/1
  Delay6/1 -> Gain8/1, Delay7/1
  Delay3/1 -> Gain5/1, Delay4/1
  Delay/1 -> Gain2/1, Delay1/1
  Delay4/1 -> Gain6/1, Delay5/1
  Delay5/1 -> Gain7/1, Delay6/1
  Signal_Input/1 -> Gain1/1, Delay/1
  Gain/1 -> Signal_Output_Mean/1
  Gain16/1 -> Add/14
  Gain14/1 -> Add/12
  Delay14/1 -> Gain18/1, Delay15/1
  Delay17/1 -> Delay18/1, Gain12/1
  Delay15/1 -> Gain19/1, Delay16/1
  Delay13/1 -> Gain17/1, Delay14/1
  Delay9/1 -> Gain13/1, Delay10/1
  Delay16/1 -> Gain20/1, Delay17/1
  Delay12/1 -> Gain16/1, Delay13/1
  Delay11/1 -> Gain15/1, Delay12/1
  Delay8/1 -> Delay9/1, Gain10/1
  Gain13/1 -> Add/11
  Gain15/1 -> Add/13
  Gain12/1 -> Add/19
  Gain19/1 -> Add/17
  Gain18/1 -> Add/16
  Gain20/1 -> Add/18
  Delay10/1 -> Gain14/1, Delay11/1
  Gain17/1 -> Add/15
  Gain11/1 -> Add/20
  Delay18/1 -> Gain11/1
  Add/1 -> Gain/1

== system LinearRegressorIP/Linear_Regression_4Taps/Running_mean_Window_4_Signal ==
  Signal_Input : Inport
  Trigger : TriggerPort  VariantControl=(inherit)  PortDimensions=1
  Add : Sum  Inputs=++++
  Delay6 : Delay  DelayLength=1
  Delay7 : Delay  DelayLength=1
  Delay8 : Delay  DelayLength=1
  Gain : Gain  Gain=1/4
  Signal_Output_Mean : Outport
  wires:
  Gain/1 -> Signal_Output_Mean/1
  Add/1 -> Gain/1
  Signal_Input/1 -> Add/1, Delay6/1
  Delay7/1 -> Add/3, Delay8/1
  Delay8/1 -> Add/4
  Delay6/1 -> Add/2, Delay7/1

== system LinearRegressorIP/Linear_Regression_4Taps/Running_mean_Window_4_SignalTimesSample ==
  Signal_Input : Inport
  Trigger : TriggerPort  VariantControl=(inherit)  PortDimensions=1
  Add : Sum  Inputs=++++
  Delay6 : Delay  DelayLength=1
  Delay7 : Delay  DelayLength=1
  Delay8 : Delay  DelayLength=1
  Gain : Gain  Gain=1/4
  Gain10 : Gain
  Gain7 : Gain  Gain=4
  Gain8 : Gain  Gain=3
  Gain9 : Gain  Gain=2
  Signal_Output_Mean : Outport
  wires:
  Add/1 -> Gain/1
  Gain10/1 -> Add/4
  Gain9/1 -> Add/3
  Gain8/1 -> Add/2
  Gain7/1 -> Add/1
  Delay7/1 -> Gain9/1, Delay8/1
  Delay6/1 -> Gain8/1, Delay7/1
  Signal_Input/1 -> Gain7/1, Delay6/1
  Delay8/1 -> Gain10/1
  Gain/1 -> Signal_Output_Mean/1

== system LinearRegressorIP/Linear_Regression_50Taps/LR_Calcer ==
  RMW_SignalTimesSample : Inport
  RMW_SignalT : Inport  Port=2
  samples_mean : Inport  Port=3
  FaktorCalcAlpha1 : Inport  Port=4
  Tabs : Inport  Port=5
  Divide : Product  Inputs=*/
  Product : Product
  Product1 : Product
  Product2 : Product
  Subtract : Sum  Inputs=+-
  Subtract2 : Sum  Inputs=-+
  Subtract3 : Sum
  Alpha_1 : Outport
  Alpha_0 : Outport  Port=2
  Signal_LR : Outport  Port=3
  wires:
  samples_mean/1 -> Product1/2, Product/2
  RMW_SignalT/1 -> Subtract2/2, Product/1
  Tabs/1 -> Product2/2
  Divide/1 -> Alpha_1/1, Product2/1, Product1/1
  Product1/1 -> Subtract2/1
  Subtract/1 -> Divide/1
  Subtract2/1 -> Alpha_0/1, Subtract3/1
  Product/1 -> Subtract/2
  RMW_SignalTimesSample/1 -> Subtract/1
  Product2/1 -> Subtract3/2
  FaktorCalcAlpha1/1 -> Divide/2
  Subtract3/1 -> Signal_LR/1

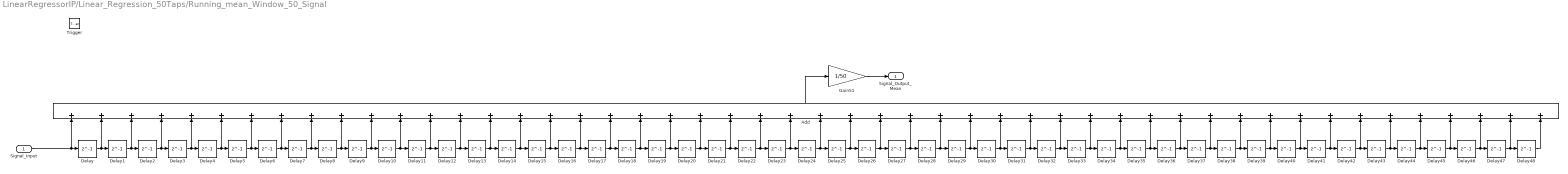
== system LinearRegressorIP/Linear_Regression_50Taps/Running_mean_Window_50_Signal ==
  Signal_Input : Inport
  Trigger : TriggerPort  VariantControl=(inherit)  PortDimensions=1
  Add : Sum  Inputs=++++++++++++++++++++++++++++++++++++++++++++++++++
  Delay{,1..48} (49 alike) : Delay  DelayLength=1
  Gain51 : Gain  Gain=1/50
  Signal_Output_Mean : Outport
  wires:
  Gain51/1 -> Signal_Output_Mean/1
  Delay30/1 -> Add/32, Delay31/1
  Delay28/1 -> Add/30, Delay29/1
  Delay27/1 -> Add/29, Delay28/1
  Delay48/1 -> Add/50
  Delay26/1 -> Add/28, Delay27/1
  Delay7/1 -> Add/9, Delay8/1
  Delay29/1 -> Add/31, Delay30/1
  Delay33/1 -> Add/35, Delay34/1
  Delay24/1 -> Add/26, Delay25/1
  Signal_Input/1 -> Add/1, Delay/1
  Delay23/1 -> Add/25, Delay24/1
  Delay22/1 -> Add/24, Delay23/1
  Delay18/1 -> Add/20, Delay19/1
  Delay21/1 -> Add/23, Delay22/1
  Delay19/1 -> Add/21, Delay20/1
  Delay17/1 -> Add/19, Delay18/1
  Delay/1 -> Add/2, Delay1/1
  Delay9/1 -> Add/11, Delay10/1
  Delay16/1 -> Add/18, Delay17/1
  Delay11/1 -> Add/13, Delay12/1
  Delay12/1 -> Add/14, Delay13/1
  Delay41/1 -> Add/43, Delay42/1
  Delay38/1 -> Add/40, Delay39/1
  Delay40/1 -> Add/42, Delay41/1
  Delay34/1 -> Add/36, Delay35/1
  Delay36/1 -> Add/38, Delay37/1
  Delay35/1 -> Add/37, Delay36/1
  Delay43/1 -> Add/45, Delay44/1
  Delay39/1 -> Add/41, Delay40/1
  Delay32/1 -> Add/34, Delay33/1
  Delay2/1 -> Add/4, Delay3/1
  Delay37/1 -> Add/39, Delay38/1
  Delay20/1 -> Add/22, Delay21/1
  Delay13/1 -> Add/15, Delay14/1
  Add/1 -> Gain51/1
  Delay8/1 -> Add/10, Delay9/1
  Delay6/1 -> Add/8, Delay7/1
  Delay4/1 -> Add/6, Delay5/1
  Delay5/1 -> Add/7, Delay6/1
  Delay3/1 -> Add/5, Delay4/1
  Delay1/1 -> Add/3, Delay2/1
  Delay42/1 -> Add/44, Delay43/1
  Delay25/1 -> Add/27, Delay26/1
  Delay44/1 -> Add/46, Delay45/1
  Delay31/1 -> Add/33, Delay32/1
  Delay14/1 -> Add/16, Delay15/1
  Delay46/1 -> Add/48, Delay47/1
  Delay10/1 -> Add/12, Delay11/1
  Delay45/1 -> Add/47, Delay46/1
  Delay47/1 -> Add/49, Delay48/1
  Delay15/1 -> Add/17, Delay16/1

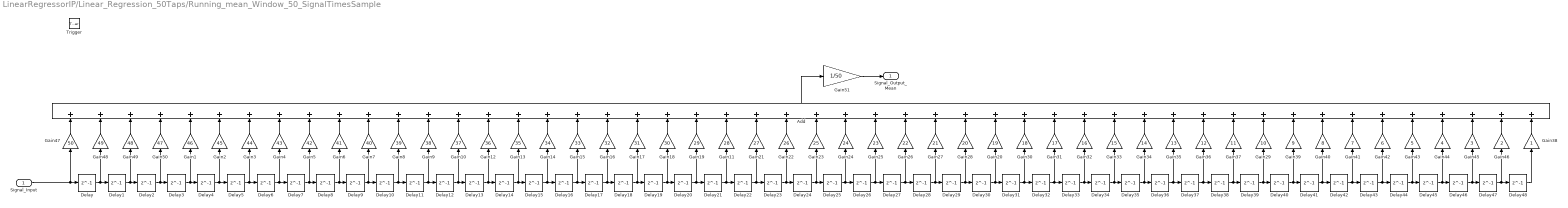
== system LinearRegressorIP/Linear_Regression_50Taps/Running_mean_Window_50_SignalTimesSample ==
  Signal_Input : Inport
  Trigger : TriggerPort  VariantControl=(inherit)  PortDimensions=1
  Add : Sum  Inputs=++++++++++++++++++++++++++++++++++++++++++++++++++
  Delay{,1..48} (49 alike) : Delay  DelayLength=1
  Gain1 : Gain  Gain=46
  Gain10 : Gain  Gain=37
  Gain11 : Gain  Gain=28
  Gain12 : Gain  Gain=36
  Gain13 : Gain  Gain=35
  Gain14 : Gain  Gain=34
  Gain15 : Gain  Gain=33
  Gain16 : Gain  Gain=32
  Gain17 : Gain  Gain=31
  Gain18 : Gain  Gain=30
  Gain19 : Gain  Gain=29
  Gain2 : Gain  Gain=45
  Gain20 : Gain  Gain=19
  Gain21 : Gain  Gain=27
  Gain22 : Gain  Gain=26
  Gain23 : Gain  Gain=25
  Gain24 : Gain  Gain=24
  Gain25 : Gain  Gain=23
  Gain26 : Gain  Gain=22
  Gain27 : Gain  Gain=21
  Gain28 : Gain  Gain=20
  Gain29 : Gain  Gain=10
  Gain3 : Gain  Gain=44
  Gain30 : Gain  Gain=18
  Gain31 : Gain  Gain=17
  Gain32 : Gain  Gain=16
  Gain33 : Gain  Gain=15
  Gain34 : Gain  Gain=14
  Gain35 : Gain  Gain=13
  Gain36 : Gain  Gain=12
  Gain37 : Gain  Gain=11
  Gain38 : Gain
  Gain39 : Gain  Gain=9
  Gain4 : Gain  Gain=43
  Gain40 : Gain  Gain=8
  Gain41 : Gain  Gain=7
  Gain42 : Gain  Gain=6
  Gain43 : Gain  Gain=5
  Gain44 : Gain  Gain=4
  Gain45 : Gain  Gain=3
  Gain46 : Gain  Gain=2
  Gain47 : Gain  Gain=50
  Gain48 : Gain  Gain=49
  Gain49 : Gain  Gain=48
  Gain5 : Gain  Gain=42
  Gain50 : Gain  Gain=47
  Gain51 : Gain  Gain=1/50
  Gain6 : Gain  Gain=41
  Gain7 : Gain  Gain=40
  Gain8 : Gain  Gain=39
  Gain9 : Gain  Gain=38
  Signal_Output_Mean : Outport
  wires:
  Signal_Input/1 -> Gain47/1, Delay/1
  Delay8/1 -> Gain6/1, Delay9/1
  Delay5/1 -> Gain3/1, Delay6/1
  Delay4/1 -> Gain2/1, Delay5/1
  Delay/1 -> Gain48/1, Delay1/1
  Delay3/1 -> Gain1/1, Delay4/1
  Delay6/1 -> Gain4/1, Delay7/1
  Delay1/1 -> Gain49/1, Delay2/1
  Delay2/1 -> Gain50/1, Delay3/1
  Delay7/1 -> Gain5/1, Delay8/1
  Gain1/1 -> Add/5
  Gain2/1 -> Add/6
  Gain3/1 -> Add/7
  Gain4/1 -> Add/8
  Gain5/1 -> Add/9
  Gain6/1 -> Add/10
  Gain7/1 -> Add/11
  Gain8/1 -> Add/12
  Gain9/1 -> Add/13
  Gain10/1 -> Add/14
  Gain11/1 -> Add/23
  Gain13/1 -> Add/16
  Gain19/1 -> Add/22
  Delay16/1 -> Gain15/1, Delay17/1
  Gain18/1 -> Add/21
  Gain14/1 -> Add/17
  Delay12/1 -> Gain10/1, Delay13/1
  Gain16/1 -> Add/19
  Gain15/1 -> Add/18
  Gain17/1 -> Add/20
  Delay11/1 -> Gain9/1, Delay12/1
  Delay10/1 -> Gain8/1, Delay11/1
  Delay15/1 -> Gain14/1, Delay16/1
  Delay9/1 -> Gain7/1, Delay10/1
  Delay14/1 -> Gain13/1, Delay15/1
  Gain12/1 -> Add/15
  Delay13/1 -> Gain12/1, Delay14/1
  Delay17/1 -> Gain16/1, Delay18/1
  Gain20/1 -> Add/32
  Gain22/1 -> Add/25
  Gain28/1 -> Add/31
  Delay25/1 -> Gain24/1, Delay26/1
  Gain27/1 -> Add/30
  Gain23/1 -> Add/26
  Delay21/1 -> Gain11/1, Delay22/1
  Gain25/1 -> Add/28
  Gain24/1 -> Add/27
  Gain26/1 -> Add/29
  Delay20/1 -> Gain19/1, Delay21/1
  Delay19/1 -> Gain18/1, Delay20/1
  Delay24/1 -> Gain23/1, Delay25/1
  Delay18/1 -> Gain17/1, Delay19/1
  Delay23/1 -> Gain22/1, Delay24/1
  Gain21/1 -> Add/24
  Delay22/1 -> Gain21/1, Delay23/1
  Delay26/1 -> Gain25/1, Delay27/1
  Gain29/1 -> Add/41
  Gain31/1 -> Add/34
  Gain37/1 -> Add/40
  Delay34/1 -> Gain33/1, Delay35/1
  Gain36/1 -> Add/39
  Gain32/1 -> Add/35
  Delay30/1 -> Gain20/1, Delay31/1
  Gain34/1 -> Add/37
  Gain33/1 -> Add/36
  Gain35/1 -> Add/38
  Delay29/1 -> Gain28/1, Delay30/1
  Delay28/1 -> Gain27/1, Delay29/1
  Delay33/1 -> Gain32/1, Delay34/1
  Delay27/1 -> Gain26/1, Delay28/1
  Delay32/1 -> Gain31/1, Delay33/1
  Gain30/1 -> Add/33
  Delay31/1 -> Gain30/1, Delay32/1
  Delay35/1 -> Gain34/1, Delay36/1
  Gain38/1 -> Add/50
  Gain40/1 -> Add/43
  Gain46/1 -> Add/49
  Delay43/1 -> Gain42/1, Delay44/1
  Gain45/1 -> Add/48
  Gain41/1 -> Add/44
  Delay39/1 -> Gain29/1, Delay40/1
  Gain43/1 -> Add/46
  Gain42/1 -> Add/45
  Gain44/1 -> Add/47
  Delay38/1 -> Gain37/1, Delay39/1
  Delay37/1 -> Gain36/1, Delay38/1
  Delay42/1 -> Gain41/1, Delay43/1
  Delay36/1 -> Gain35/1, Delay37/1
  Delay41/1 -> Gain40/1, Delay42/1
  Gain39/1 -> Add/42
  Delay40/1 -> Gain39/1, Delay41/1
  Delay44/1 -> Gain43/1, Delay45/1
  Delay48/1 -> Gain38/1
  Delay45/1 -> Gain44/1, Delay46/1
  Delay46/1 -> Gain45/1, Delay47/1
  Delay47/1 -> Gain46/1, Delay48/1
  Gain50/1 -> Add/4
  Gain49/1 -> Add/3
  Gain48/1 -> Add/2
  Gain47/1 -> Add/1
  Gain51/1 -> Signal_Output_Mean/1
  Add/1 -> Gain51/1
